simulink model "Consolidate_Observer_based_state_feedback_xfer"  (Simulink 8.6)
settings: Solver=ode45  StartTime=0.0  StopTime=6  MaxStep=.00001  RelTol=1e-3
values from neighbouring files (symbols this model uses):
  A = [0 1; -50 -15]    [consolidated_models.m]
  B = [0;1]    [consolidated_models.m]
  C = [1 0]    [consolidated_models.m]
  K = acker(A, B, [-20 -25])    [consolidated_models.m]
  L = acker(A', C', [-50, -60])'    [consolidated_models.m]
settings Model: Creator=DR_C  LastModifiedBy=DR_C
settings DebuggingCC: FcnCallInpInsideContextMsg=EnableAllAsWarning
settings GRTTargetCC: CombineOutputUpdateFcns=on  GRTInterface=off

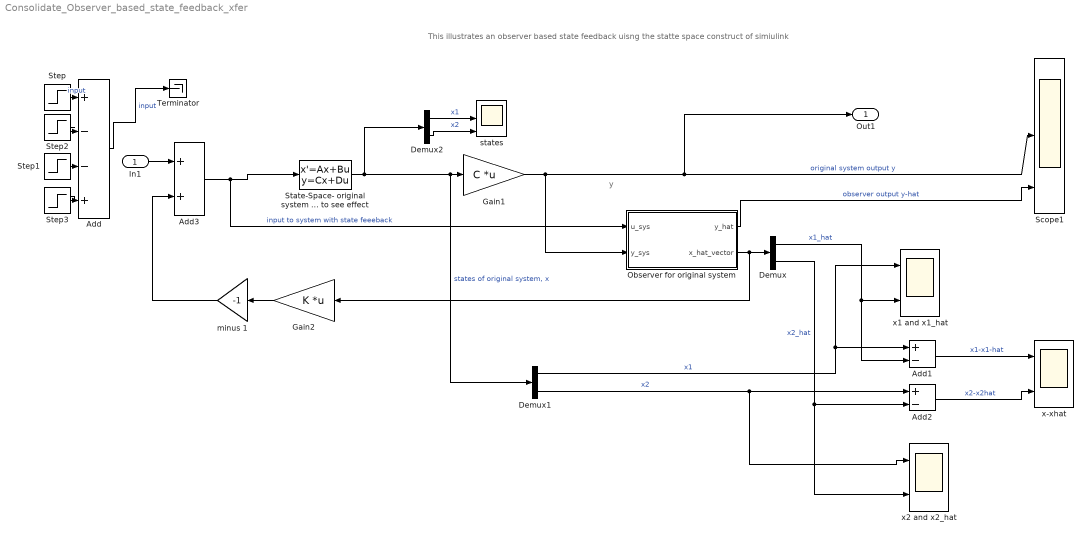
== system Consolidate_Observer_based_state_feedback_xfer ==
  note: y
  note: This illustrates an observer based state feedback uisng the statte space construct of simiulink
  In1 : Inport
  Add : Sum  Inputs=+--+
  Add1 : Sum  Inputs=+-
  Add2 : Sum  Inputs=+-
  Add3 : Sum
  Demux : Demux  Outputs=2
  Demux1 : Demux  Outputs=2
  Demux2 : Demux  Outputs=2
  Gain1 : Gain  Gain=C  Multiplication=Matrix(K*u) (u vector)
  Gain2 : Gain  Gain=K  Multiplication=Matrix(K*u) (u vector)
  Observer for original system : Subsystem
  Scope1 : Scope  NumInputPorts=3
  State-Space- original system note you can change IC's to see effect : StateSpace  A=A  B=B  C=eye(2)  D=[0;0]  X0=0
  Step : Step  Time=0  After=3  SampleTime=0
  Step1 : Step  Time=3.5  After=3  SampleTime=0
  Step2 : Step  Time=2  After=3  SampleTime=0
  Step3 : Step  Time=4.5  After=3  SampleTime=0
  Terminator : Terminator
  minus 1 : Gain  Gain=-1
  states : Scope  NumInputPorts=3
  x-xhat : Scope  NumInputPorts=2
  x1 and x1_hat : Scope  NumInputPorts=2
  x2 and x2_hat : Scope  NumInputPorts=2
  Out1 : Outport
  wires:
  State-Space- original system note you can change IC's to see effect/1 -> Gain1/1, Demux1/1, Demux2/1  "states of original system, x"
  Observer for original system/1(y_hat) -> Scope1/3  "observer output y-hat"
  Gain1/1 -> Observer for original system/2(y_sys), Scope1/2, Out1/1  "original system output y"
  Observer for original system/2(x_hat_vector) -> Demux/1, Gain2/1
  Demux1/1 -> x1 and x1_hat/1, Add1/1  "x1"
  Demux/1 -> x1 and x1_hat/2, Add1/2  "x1_hat"
  Demux1/2 -> x2 and x2_hat/1, Add2/1  "x2"
  Demux/2 -> x2 and x2_hat/2, Add2/2  "x2_hat"
  Step/1 -> Add/1  "input"
  Step2/1 -> Add/2
  Demux2/2 -> states/3  "x2"
  Demux2/1 -> states/2  "x1"
  Step1/1 -> Add/3
  Step3/1 -> Add/4
  Add1/1 -> x-xhat/1  "x1-x1-hat"
  Add2/1 -> x-xhat/2  "x2-x2hat"
  Gain2/1 -> minus 1/1
  minus 1/1 -> Add3/2
  Add3/1 -> State-Space- original system note you can change IC's to see effect/1, Observer for original system/1(u_sys)  "input to system with state feeeback"
  In1/1 -> Add3/1
  Add/1 -> Terminator/1  "input"

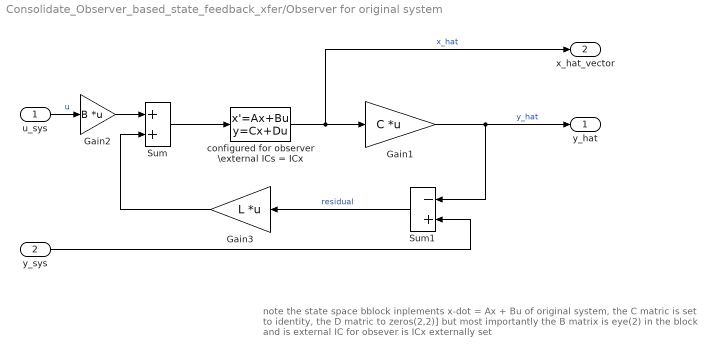
== system Consolidate_Observer_based_state_feedback_xfer/Observer for original system ==
  note: note the state space bblock
      | inplements x-dot = Ax + Bu of original
      | system, the C matric is set to identity, the D matric to zeros(2,2)] but most importantly
      | the B matrix is eye(2) in the block and is external
      |
      | IC for obsever is ICx externally set
  u_sys : Inport
  y_sys : Inport  Port=2
  Gain1 : Gain  Gain=C  Multiplication=Matrix(K*u) (u vector)
  Gain2 : Gain  Gain=B  Multiplication=Matrix(K*u)
  Gain3 : Gain  Gain=L  Multiplication=Matrix(K*u)
  Sum : Sum
  Sum1 : Sum  Inputs=-+
  configured for observer \external ICs = ICx : StateSpace  A=A  B=eye(2)  C=eye(2)  D=zeros(2,2)  X0=0
  y_hat : Outport
  x_hat_vector : Outport  Port=2
  wires:
  Sum/1 -> configured for observer \external ICs = ICx/1
  configured for observer \external ICs = ICx/1 -> Gain1/1, x_hat_vector/1  "x_hat"
  u_sys/1 -> Gain2/1  "u"
  Gain1/1 -> y_hat/1, Sum1/1  "y_hat"
  Gain2/1 -> Sum/1
  Gain3/1 -> Sum/2
  Sum1/1 -> Gain3/1  "residual"
  y_sys/1 -> Sum1/2
